simulink model "Att_project_simulink"  (R2022b)
settings: Solver=ode8  StartTime=0.0  StopTime=5000  FixedStep=0.5  RelTol=1e-9  AbsTol=1e-9
values from neighbouring files (symbols this model uses):
  A_R = A_R_BL * ALN_R    [Attitude_proj.m]
  A_T = A_R_BL    [Attitude_proj.m]
  accuracy_earth = deg2rad(10/60)    [Attitude_proj.m]
  accuracy_mag = deg2rad(300/60)    [Attitude_proj.m]
  Cd = 2.3    [Attitude_proj.m]
  I = [Ix 0 0; 0 Iy 0 ; 0 0 Iz]    [Attitude_proj.m]
  Ix = 0.07    [Attitude_proj.m]
  Iy = 0.0504    [Attitude_proj.m]
  Iz = 0.0109    [Attitude_proj.m]
  kd_detum = 2 .* kp_detum    [Attitude_proj.m]
  kd_slew = 2 * kp_slew    [Attitude_proj.m]
  kd_track = kd_detum    [Attitude_proj.m]
  kp_detum = [0.00008 0.0005 0.0005]    [Attitude_proj.m]
  kp_slew = [0.0005 0.0004 0.0004]    [Attitude_proj.m]
  kp_track = kp_detum    [Attitude_proj.m]
  Kx = (Iy-Iz)/Ix    (= 0.564285714286)    [Attitude_proj.m]
  Ky = (Iz-Ix)/Iy    (= -1.17261904762)    [Attitude_proj.m]
  Kz = (Ix-Iy)/Iz    (= 1.79816513761)    [Attitude_proj.m]
  m_para = [0.03;0.04;0.05]    [Attitude_proj.m]
  ortog = (1/3 * deg2rad(1)^2)    [Attitude_proj.m]
  P = Fe/c    (= 4.52980041279e-06)    [Attitude_proj.m]
  q_r = [q1r q2r q3r q4r]    [Attitude_proj.m]
  rho_d_main = 0.1    [Attitude_proj.m]
  rho_d_panel = 0.1    [Attitude_proj.m]
  rho_s_main = 0.5    [Attitude_proj.m]
  rho_s_panel = 0.1    [Attitude_proj.m]
  Rs = 147098074    [Attitude_proj.m]
  w0x = 0.0001    [Attitude_proj.m]
  w0y = orbit.n + 0.005    [Attitude_proj.m]
  w0z = 0.0002    [Attitude_proj.m]
  w_track = [0; orbit.n ; 0]    [Attitude_proj.m]
  zero_w = [ 0; 0; 0]    [Attitude_proj.m]
undefined symbols (not defined in the file or in its folder): body, DiscIntNeverNeededParam, g, h, K, k2, magnitude, orbit, phi0, psi0, theta0, thrus
libraries: vrlib x60, matrix_library x7, simulink x4, sharedutil x4, simulink_extras x2, cstblocks x1, aerolibconvert2 x1, sharedtransform x1
(part 2 of 2)

== system Att_project_simulink/Kynematics/Quaternions ==
  wB : Inport
  Demux : Demux  Outputs=3
  Determinant of 3x3 Matrix : sharedutil/Determinant of 3x3 Matrix  aMode=aMode
  Gain : Gain  Gain=-1
  Gain1 : Gain  Gain=-1
  Gain2 : Gain  Gain=-1
  Gain3 : Gain  Gain=0.5
  Ground{,1..3} (4 alike) : Ground
  Integrator : Integrator  InitialCondition=q_r
  MatrixMultiply : Product  Multiplication=Matrix(*)
  Quaternions to Direction Cosine Matrix : sharedtransform/Quaternions to  Direction Cosine Matrix  aMode=aMode
  Reshape : Reshape  OutputDimensionality=Customize  OutputDimensions=[4,4]
  Scope : Scope
  Scope1 : Scope
  Scope2 : Scope
  To Workspace : ToWorkspace  VariableName=quaternions  SaveFormat=Timeseries  SampleTime=-1
  Vector Concatenate : Concatenate  NumInputs=16
  q(t) : Outport
  tag scope: q=global
  wires:
  wB/1 -> Demux/1
  Ground3/1 -> Vector Concatenate/1
  Ground2/1 -> Vector Concatenate/6
  Ground1/1 -> Vector Concatenate/16
  Ground/1 -> Vector Concatenate/11
  Demux/1 -> Vector Concatenate/13, Vector Concatenate/10, Gain/1  "w_x"
  Demux/2 -> Vector Concatenate/3, Vector Concatenate/14, Gain1/1  "w_y"
  Demux/3 -> Vector Concatenate/5, Gain2/1, Vector Concatenate/15  "w_z"
  Gain2/1 -> Vector Concatenate/12, Vector Concatenate/2
  Gain/1 -> Vector Concatenate/4, Vector Concatenate/7
  Gain1/1 -> Vector Concatenate/9, Vector Concatenate/8
  Vector Concatenate/1 -> Reshape/1
  Reshape/1 -> Gain3/1  "Omega"
  Gain3/1 -> MatrixMultiply/1
  MatrixMultiply/1 -> Integrator/1
  Integrator/1 -> q(t)/1, Quaternions to Direction Cosine Matrix/1, [q], To Workspace/1, Scope/1, MatrixMultiply/2  "q(t)"
  Quaternions to Direction Cosine Matrix/1 -> Determinant of 3x3 Matrix/1, Scope1/1
  Determinant of 3x3 Matrix/1 -> Scope2/1

== system Att_project_simulink/Attitude determination/Triad Method/Error ==
  A_err : Inport
  Acos2 : Trigonometry  Operator=acos
  Constant6 : Constant
  Extract Diagonal3 : matrix_library/Extract Diagonal
      settings: LibrarySourceBlock=|
      | simulink/Matrix
      | Operations/Extract Diagonal
  Gain2 : Gain  Gain=0.5
  Radians to Degrees2 : simulink_extras/Transformations/Radians to Degrees
  Sum of Elements3 : Sum  Inputs=+
  Sum7 : Sum  Inputs=|+-
  error : Outport
  wires:
  Extract Diagonal3/1 -> Sum of Elements3/1
  Acos2/1 -> Radians to Degrees2/1
  Sum of Elements3/1 -> Sum7/1
  Radians to Degrees2/1 -> error/1
  A_err/1 -> Extract Diagonal3/1
  Sum7/1 -> Gain2/1
  Constant6/1 -> Sum7/2
  Gain2/1 -> Acos2/1

== system Att_project_simulink/Attitude determination/Triad Method/Error1 ==
  Id : Inport
  Acos2 : Trigonometry  Operator=acos
  Constant6 : Constant
  Extract Diagonal3 : matrix_library/Extract Diagonal
      settings: LibrarySourceBlock=|
      | simulink/Matrix
      | Operations/Extract Diagonal
  Gain2 : Gain  Gain=0.5
  Radians to Degrees2 : simulink_extras/Transformations/Radians to Degrees
  Sum of Elements3 : Sum  Inputs=+
  Sum7 : Sum  Inputs=|+-
  error : Outport
  wires:
  Gain2/1 -> Acos2/1
  Constant6/1 -> Sum7/2
  Sum7/1 -> Gain2/1
  Id/1 -> Extract Diagonal3/1
  Radians to Degrees2/1 -> error/1
  Sum of Elements3/1 -> Sum7/1
  Acos2/1 -> Radians to Degrees2/1
  Extract Diagonal3/1 -> Sum of Elements3/1

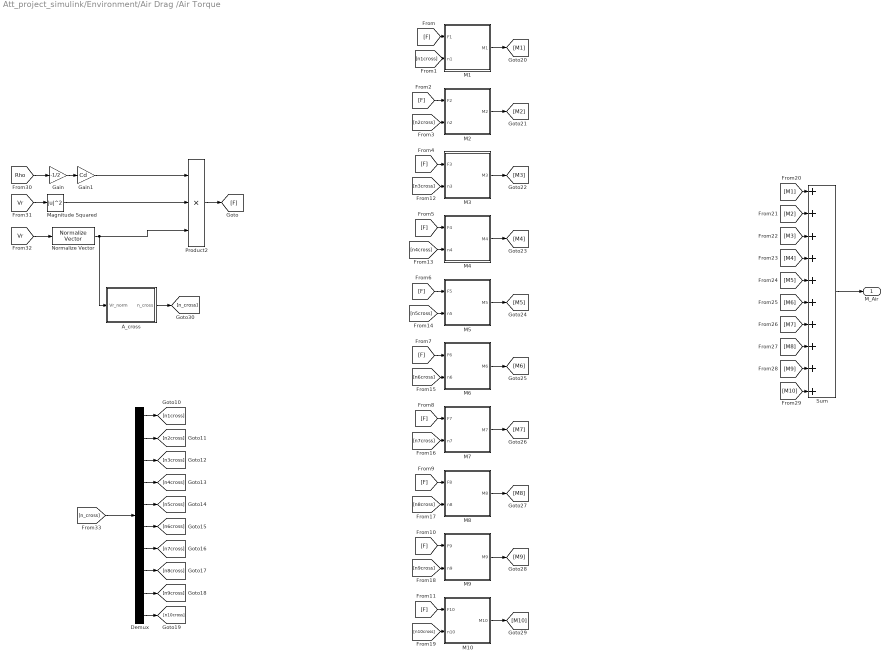
== system Att_project_simulink/Environment/Air Drag /Air Torque ==
  A_cross : Subsystem
  Demux : Demux  Outputs=10
  Gain : Gain  Gain=-1/2
  Gain1 : Gain  Gain=Cd
  M1 : Subsystem
  M10 : Subsystem
  M2 : Subsystem
  M3 : Subsystem
  M4 : Subsystem
  M5 : Subsystem
  M6 : Subsystem
  M7 : Subsystem
  M8 : Subsystem
  M9 : Subsystem
  Magnitude Squared : Math  Operator=magnitude^2
  Normalize Vector : vrlib/Utilities/Normalize Vector  maxzero=0
  Product2 : Product  Inputs=3
  Sum : Sum  Inputs=++++++++++
  M_Air : Outport
  wires:
  [n_cross] -> Demux/1
  Demux/1 -> [n1cross]
  Demux/2 -> [n2cross]
  Demux/3 -> [n3cross]
  Demux/4 -> [n4cross]
  Demux/5 -> [n5cross]
  Demux/6 -> [n6cross]
  Demux/7 -> [n7cross]
  Demux/8 -> [n8cross]
  Demux/9 -> [n9cross]
  Demux/10 -> [n10cross]
  [F] -> M1/1(F1)
  [n1cross] -> M1/2(n1)
  [F] -> M2/1(F2)
  [F] -> M10/1(F10)
  [F] -> M9/1(F9)
  [F] -> M8/1(F8)
  [F] -> M7/1(F7)
  [F] -> M6/1(F6)
  [F] -> M5/1(F5)
  [F] -> M4/1(F4)
  [F] -> M3/1(F3)
  [n3cross] -> M3/2(n3)
  [n4cross] -> M4/2(n4)
  [n5cross] -> M5/2(n5)
  [n6cross] -> M6/2(n6)
  [n7cross] -> M7/2(n7)
  [n8cross] -> M8/2(n8)
  [n9cross] -> M9/2(n9)
  [n10cross] -> M10/2(n10)
  [n2cross] -> M2/2(n2)
  M1/1(M1) -> [M1]
  M2/1(M2) -> [M2]
  M3/1(M3) -> [M3]
  M4/1(M4) -> [M4]
  M5/1(M5) -> [M5]
  M6/1(M6) -> [M6]
  M7/1(M7) -> [M7]
  M8/1(M8) -> [M8]
  M9/1(M9) -> [M9]
  M10/1(M10) -> [M10]
  [M1] -> Sum/1
  [M2] -> Sum/2
  [M3] -> Sum/3
  [M4] -> Sum/4
  [M5] -> Sum/5
  [M6] -> Sum/6
  [M7] -> Sum/7
  [M8] -> Sum/8
  [M9] -> Sum/9
  [M10] -> Sum/10
  Sum/1 -> M_Air/1
  [Rho] -> Gain/1
  A_cross/1(n_cross) -> [n_cross]
  Gain/1 -> Gain1/1
  Gain1/1 -> Product2/1
  Magnitude Squared/1 -> Product2/2
  [Vr] -> Magnitude Squared/1
  Product2/1 -> [F]
  [Vr] -> Normalize Vector/1
  Normalize Vector/1 -> A_cross/1(Vr_norm), Product2/3

== system Att_project_simulink/Environment/Magnetif Field Model/Ground Track ==
  Rn : Inport
  ThetaG0 : Inport  Port=2
  t : Inport  Port=3
  W_E : Inport  Port=4
  t0 : Inport  Port=5
  Asin : Trigonometry  Operator=asin
  Atan2 : Trigonometry  Operator=atan2
  Divide : Product  Inputs=*/
  Math Function : Math  Operator=square  SignedPower=on
  Math Function1 : Math  Operator=sqrt  SignedPower=on
  Product : Product
  Selector : Selector  InputPortWidth=3  IndexOptions=Index vector (dialog)  Indices=[3]  OutputSizes=1
  Selector1 : Selector  InputPortWidth=3  IndexOptions=Index vector (dialog)  Indices=[2]  OutputSizes=1
  Selector2 : Selector  InputPortWidth=3  IndexOptions=Index vector (dialog)  Indices=[1 ]  OutputSizes=1
  Sum : Sum  Inputs=|+-
  Sum of Elements : Sum  Inputs=+
  Sum1 : Sum  Inputs=|++
  Sum2 : Sum  Inputs=|+-
  Lon : Outport
  Lat : Outport  Port=2
  R_norm : Outport  Port=3
  wires:
  Rn/1 -> Selector2/1, Selector1/1, Math Function/1, Selector/1
  Selector/1 -> Divide/1
  Math Function1/1 -> R_norm/1, Divide/2
  Divide/1 -> Asin/1
  Asin/1 -> Lat/1
  Selector1/1 -> Atan2/1
  Selector2/1 -> Atan2/2
  t/1 -> Sum/1
  t0/1 -> Sum/2
  Sum/1 -> Product/1
  W_E/1 -> Product/2
  Product/1 -> Sum1/1
  ThetaG0/1 -> Sum1/2
  Sum1/1 -> Sum2/2  "ThetaG"
  Atan2/1 -> Sum2/1
  Sum2/1 -> Lon/1
  Math Function/1 -> Sum of Elements/1
  Sum of Elements/1 -> Math Function1/1

== system Att_project_simulink/Environment/SRP/F1 ==
  In1 : Inport
  Input : Inport  Port=2
  Constant : Constant  Value=-P
  Constant1 : Constant  Value=body.A1
  Constant2 : Constant
  Constant3 : Constant  Value=body.r1
  Constant6 : Constant  Value=rho_s_main
  Constant7 : Constant  Value=(2/3)*rho_d_main
  Cross Product : vrlib/Utilities/Cross Product
  Dot Product : DotProduct  OutDataTypeStr=Inherit: Inherit via internal rule
  Dot Product1 : DotProduct  OutDataTypeStr=Inherit: Inherit via internal rule
  Gain3 : Gain  Gain=2*rho_s_main
  Normalize Vector : vrlib/Utilities/Normalize Vector  maxzero=0
  Normalize Vector1 : vrlib/Utilities/Normalize Vector  maxzero=0
  Normalize Vector2 : vrlib/Utilities/Normalize Vector  maxzero=0
  Product : Product  Inputs=3
  Product1 : Product
  Product2 : Product
  Product3 : Product
  Sum : Sum  Inputs=+-
  Sum1 : Sum
  Sum2 : Sum  Inputs=|++
  Switch : Switch  Criteria=u2 > Threshold  SaturateOnIntegerOverflow=off  InputSameDT=off
  Zero : Constant  Value=0  OutDataTypeStr=Inherit: Inherit via back propagation
  T1 : Outport
  wires:
  Dot Product/1 -> Product/3
  Sum1/1 -> Product3/2
  Product2/1 -> Sum1/2
  Constant2/1 -> Sum/1
  [n1] -> Dot Product1/2
  Constant6/1 -> Sum/2
  Sum2/1 -> Product2/2
  Gain3/1 -> Sum2/1
  Constant7/1 -> Sum2/2
  Product1/1 -> Sum1/1
  Sum/1 -> Product1/1
  [n1] -> Product2/1
  Product/1 -> Product3/1
  Constant1/1 -> Product/2
  [n1] -> Dot Product/2
  Constant/1 -> Product/1
  In1/1 -> [n1]
  Input/1 -> [Sb]
  Dot Product1/1 -> [Sb_dot_N1], Gain3/1
  [Sb_dot_N1] -> Switch/2
  Zero/1 -> Switch/3
  Product3/1 -> Switch/1
  Switch/1 -> Cross Product/1
  Constant3/1 -> Cross Product/2
  Cross Product/1 -> T1/1
  [Sb] -> Normalize Vector/1
  Normalize Vector/1 -> Dot Product/1
  [Sb] -> Normalize Vector1/1
  Normalize Vector1/1 -> Product1/2
  [Sb] -> Normalize Vector2/1
  Normalize Vector2/1 -> Dot Product1/1

== system Att_project_simulink/Environment/SRP/F10 ==
  In1 : Inport
  In2 : Inport  Port=2
  Constant10 : Constant
  Constant11 : Constant  Value=rho_s_panel
  Constant12 : Constant  Value=(2/3)*rho_d_panel
  Constant3 : Constant  Value=body.r10
  Constant8 : Constant  Value=-P
  Constant9 : Constant  Value=body.A10
  Cross Product : vrlib/Utilities/Cross Product
  Dot Product2 : DotProduct  OutDataTypeStr=Inherit: Inherit via internal rule
  Dot Product3 : DotProduct  OutDataTypeStr=Inherit: Inherit via internal rule
  Gain4 : Gain  Gain=2*rho_s_panel
  Normalize Vector : vrlib/Utilities/Normalize Vector  maxzero=0
  Normalize Vector1 : vrlib/Utilities/Normalize Vector  maxzero=0
  Normalize Vector2 : vrlib/Utilities/Normalize Vector  maxzero=0
  Product3 : Product
  Product4 : Product  Inputs=3
  Product5 : Product
  Product6 : Product
  Sum3 : Sum  Inputs=+-
  Sum4 : Sum
  Sum5 : Sum  Inputs=|++
  Switch : Switch  Criteria=u2 > Threshold  SaturateOnIntegerOverflow=off  InputSameDT=off
  Zero : Constant  Value=0  OutDataTypeStr=Inherit: Inherit via back propagation
  T10 : Outport
  wires:
  Product6/1 -> Sum4/2
  Constant9/1 -> Product4/2
  Gain4/1 -> Sum5/1
  Dot Product2/1 -> Product4/3
  [n10] -> Dot Product2/2
  Sum3/1 -> Product5/1
  Constant11/1 -> Sum3/2
  Constant8/1 -> Product4/1
  Sum5/1 -> Product6/2
  Product4/1 -> Product3/1
  Constant12/1 -> Sum5/2
  [n10] -> Product6/1
  Product5/1 -> Sum4/1
  [n10] -> Dot Product3/2
  Dot Product3/1 -> [Sb_dot_N10], Gain4/1
  Constant10/1 -> Sum3/1
  Sum4/1 -> Product3/2
  In1/1 -> [n10]
  In2/1 -> [Sb]
  Cross Product/1 -> T10/1
  Constant3/1 -> Cross Product/2
  Product3/1 -> Switch/1
  [Sb_dot_N10] -> Switch/2
  Switch/1 -> Cross Product/1
  Zero/1 -> Switch/3
  [Sb] -> Normalize Vector/1
  Normalize Vector/1 -> Dot Product2/1
  [Sb] -> Normalize Vector1/1
  Normalize Vector1/1 -> Product5/2
  [Sb] -> Normalize Vector2/1
  Normalize Vector2/1 -> Dot Product3/1

== system Att_project_simulink/Environment/SRP/F2 ==
  In1 : Inport
  In2 : Inport  Port=2
  Constant10 : Constant
  Constant11 : Constant  Value=rho_s_main
  Constant12 : Constant  Value=(2/3)*rho_d_main
  Constant3 : Constant  Value=body.r2
  Constant8 : Constant  Value=-P
  Constant9 : Constant  Value=body.A2
  Cross Product : vrlib/Utilities/Cross Product
  Dot Product2 : DotProduct  OutDataTypeStr=Inherit: Inherit via internal rule
  Dot Product3 : DotProduct  OutDataTypeStr=Inherit: Inherit via internal rule
  Gain4 : Gain  Gain=2*rho_s_main
  Normalize Vector : vrlib/Utilities/Normalize Vector  maxzero=0
  Normalize Vector1 : vrlib/Utilities/Normalize Vector  maxzero=0
  Normalize Vector2 : vrlib/Utilities/Normalize Vector  maxzero=0
  Product3 : Product
  Product4 : Product  Inputs=3
  Product5 : Product
  Product6 : Product
  Sum3 : Sum  Inputs=+-
  Sum4 : Sum
  Sum5 : Sum  Inputs=|++
  Switch : Switch  Criteria=u2 > Threshold  SaturateOnIntegerOverflow=off  InputSameDT=off
  Zero : Constant  Value=0  OutDataTypeStr=Inherit: Inherit via back propagation
  T2 : Outport
  wires:
  Product6/1 -> Sum4/2
  Constant9/1 -> Product4/2
  Gain4/1 -> Sum5/1
  Dot Product2/1 -> Product4/3
  [n2] -> Dot Product2/2
  Sum3/1 -> Product5/1
  Constant11/1 -> Sum3/2
  Constant8/1 -> Product4/1
  Sum5/1 -> Product6/2
  Product4/1 -> Product3/1
  Constant12/1 -> Sum5/2
  [n2] -> Product6/1
  Product5/1 -> Sum4/1
  [n2] -> Dot Product3/2
  Dot Product3/1 -> [Sb_dot_N2], Gain4/1
  Constant10/1 -> Sum3/1
  Sum4/1 -> Product3/2
  In1/1 -> [n2]
  In2/1 -> [Sb]
  Cross Product/1 -> T2/1
  Constant3/1 -> Cross Product/2
  Product3/1 -> Switch/1
  [Sb_dot_N2] -> Switch/2
  Switch/1 -> Cross Product/1
  Zero/1 -> Switch/3
  [Sb] -> Normalize Vector/1
  Normalize Vector/1 -> Dot Product2/1
  [Sb] -> Normalize Vector1/1
  Normalize Vector1/1 -> Product5/2
  [Sb] -> Normalize Vector2/1
  Normalize Vector2/1 -> Dot Product3/1

== system Att_project_simulink/Environment/SRP/F3 ==
  In1 : Inport
  In2 : Inport  Port=2
  Constant10 : Constant
  Constant11 : Constant  Value=rho_s_main
  Constant12 : Constant  Value=(2/3)*rho_d_main
  Constant3 : Constant  Value=body.r3
  Constant8 : Constant  Value=-P
  Constant9 : Constant  Value=body.A3
  Cross Product : vrlib/Utilities/Cross Product
  Dot Product2 : DotProduct  OutDataTypeStr=Inherit: Inherit via internal rule
  Dot Product3 : DotProduct  OutDataTypeStr=Inherit: Inherit via internal rule
  Gain4 : Gain  Gain=2*rho_s_main
  Normalize Vector : vrlib/Utilities/Normalize Vector  maxzero=0
  Normalize Vector1 : vrlib/Utilities/Normalize Vector  maxzero=0
  Normalize Vector2 : vrlib/Utilities/Normalize Vector  maxzero=0
  Product3 : Product
  Product4 : Product  Inputs=3
  Product5 : Product
  Product6 : Product
  Sum3 : Sum  Inputs=+-
  Sum4 : Sum
  Sum5 : Sum  Inputs=|++
  Switch : Switch  Criteria=u2 > Threshold  SaturateOnIntegerOverflow=off  InputSameDT=off
  Zero : Constant  Value=0  OutDataTypeStr=Inherit: Inherit via back propagation
  T3 : Outport
  wires:
  Product6/1 -> Sum4/2
  Constant9/1 -> Product4/2
  Gain4/1 -> Sum5/1
  Dot Product2/1 -> Product4/3
  [n3] -> Dot Product2/2
  Sum3/1 -> Product5/1
  Constant11/1 -> Sum3/2
  Constant8/1 -> Product4/1
  Sum5/1 -> Product6/2
  Product4/1 -> Product3/1
  Constant12/1 -> Sum5/2
  [n3] -> Product6/1
  Product5/1 -> Sum4/1
  [n3] -> Dot Product3/2
  Dot Product3/1 -> [Sb_dot_N3], Gain4/1
  Constant10/1 -> Sum3/1
  Sum4/1 -> Product3/2
  In1/1 -> [n3]
  In2/1 -> [Sb]
  Cross Product/1 -> T3/1
  Constant3/1 -> Cross Product/2
  Product3/1 -> Switch/1
  [Sb_dot_N3] -> Switch/2
  Switch/1 -> Cross Product/1
  Zero/1 -> Switch/3
  Normalize Vector/1 -> Dot Product2/1
  [Sb] -> Normalize Vector/1
  Normalize Vector1/1 -> Product5/2
  [Sb] -> Normalize Vector1/1
  [Sb] -> Normalize Vector2/1
  Normalize Vector2/1 -> Dot Product3/1

== system Att_project_simulink/Environment/SRP/F4 ==
  In1 : Inport
  In2 : Inport  Port=2
  Constant10 : Constant
  Constant11 : Constant  Value=rho_s_main
  Constant12 : Constant  Value=(2/3)*rho_d_main
  Constant3 : Constant  Value=body.r4
  Constant8 : Constant  Value=-P
  Constant9 : Constant  Value=body.A4
  Cross Product : vrlib/Utilities/Cross Product
  Dot Product2 : DotProduct  OutDataTypeStr=Inherit: Inherit via internal rule
  Dot Product3 : DotProduct  OutDataTypeStr=Inherit: Inherit via internal rule
  Gain4 : Gain  Gain=2*rho_s_main
  Normalize Vector : vrlib/Utilities/Normalize Vector  maxzero=0
  Normalize Vector1 : vrlib/Utilities/Normalize Vector  maxzero=0
  Normalize Vector2 : vrlib/Utilities/Normalize Vector  maxzero=0
  Product3 : Product
  Product4 : Product  Inputs=3
  Product5 : Product
  Product6 : Product
  Sum3 : Sum  Inputs=+-
  Sum4 : Sum
  Sum5 : Sum  Inputs=|++
  Switch : Switch  Criteria=u2 > Threshold  SaturateOnIntegerOverflow=off  InputSameDT=off
  Zero : Constant  Value=0  OutDataTypeStr=Inherit: Inherit via back propagation
  T4 : Outport
  wires:
  Product6/1 -> Sum4/2
  Constant9/1 -> Product4/2
  Gain4/1 -> Sum5/1
  Dot Product2/1 -> Product4/3
  [n4] -> Dot Product2/2
  Sum3/1 -> Product5/1
  Constant11/1 -> Sum3/2
  Constant8/1 -> Product4/1
  Sum5/1 -> Product6/2
  Product4/1 -> Product3/1
  Constant12/1 -> Sum5/2
  [n4] -> Product6/1
  Product5/1 -> Sum4/1
  [n4] -> Dot Product3/2
  Dot Product3/1 -> [Sb_dot_N4], Gain4/1
  Constant10/1 -> Sum3/1
  Sum4/1 -> Product3/2
  In1/1 -> [n4]
  In2/1 -> [Sb]
  Cross Product/1 -> T4/1
  Constant3/1 -> Cross Product/2
  Product3/1 -> Switch/1
  [Sb_dot_N4] -> Switch/2
  Switch/1 -> Cross Product/1
  Zero/1 -> Switch/3
  [Sb] -> Normalize Vector/1
  Normalize Vector/1 -> Dot Product2/1
  [Sb] -> Normalize Vector1/1
  Normalize Vector1/1 -> Product5/2
  [Sb] -> Normalize Vector2/1
  Normalize Vector2/1 -> Dot Product3/1

== system Att_project_simulink/Environment/SRP/F5 ==
  In1 : Inport
  In2 : Inport  Port=2
  Constant10 : Constant
  Constant11 : Constant  Value=rho_s_main
  Constant12 : Constant  Value=(2/3)*rho_d_main
  Constant3 : Constant  Value=body.r5
  Constant8 : Constant  Value=-P
  Constant9 : Constant  Value=body.A5
  Cross Product : vrlib/Utilities/Cross Product
  Dot Product2 : DotProduct  OutDataTypeStr=Inherit: Inherit via internal rule
  Dot Product3 : DotProduct  OutDataTypeStr=Inherit: Inherit via internal rule
  Gain4 : Gain  Gain=2*rho_s_main
  Normalize Vector : vrlib/Utilities/Normalize Vector  maxzero=0
  Normalize Vector1 : vrlib/Utilities/Normalize Vector  maxzero=0
  Normalize Vector2 : vrlib/Utilities/Normalize Vector  maxzero=0
  Product3 : Product
  Product4 : Product  Inputs=3
  Product5 : Product
  Product6 : Product
  Sum3 : Sum  Inputs=+-
  Sum4 : Sum
  Sum5 : Sum  Inputs=|++
  Switch : Switch  Criteria=u2 > Threshold  SaturateOnIntegerOverflow=off  InputSameDT=off
  Zero : Constant  Value=0  OutDataTypeStr=Inherit: Inherit via back propagation
  T5 : Outport
  wires:
  Product6/1 -> Sum4/2
  Constant9/1 -> Product4/2
  Gain4/1 -> Sum5/1
  Dot Product2/1 -> Product4/3
  [n5] -> Dot Product2/2
  Sum3/1 -> Product5/1
  Constant11/1 -> Sum3/2
  Constant8/1 -> Product4/1
  Sum5/1 -> Product6/2
  Product4/1 -> Product3/1
  Constant12/1 -> Sum5/2
  [n5] -> Product6/1
  Product5/1 -> Sum4/1
  [n5] -> Dot Product3/2
  Dot Product3/1 -> [Sb_dot_N5], Gain4/1
  Constant10/1 -> Sum3/1
  Sum4/1 -> Product3/2
  In1/1 -> [n5]
  In2/1 -> [Sb]
  Cross Product/1 -> T5/1
  Constant3/1 -> Cross Product/2
  Product3/1 -> Switch/1
  [Sb_dot_N5] -> Switch/2
  Switch/1 -> Cross Product/1
  Zero/1 -> Switch/3
  [Sb] -> Normalize Vector/1
  Normalize Vector/1 -> Dot Product2/1
  [Sb] -> Normalize Vector1/1
  Normalize Vector1/1 -> Product5/2
  [Sb] -> Normalize Vector2/1
  Normalize Vector2/1 -> Dot Product3/1

== system Att_project_simulink/Environment/SRP/F6 ==
  In1 : Inport
  In2 : Inport  Port=2
  Constant10 : Constant
  Constant11 : Constant  Value=rho_s_main
  Constant12 : Constant  Value=(2/3)*rho_d_main
  Constant3 : Constant  Value=body.r6
  Constant8 : Constant  Value=-P
  Constant9 : Constant  Value=body.A6
  Cross Product : vrlib/Utilities/Cross Product
  Dot Product2 : DotProduct  OutDataTypeStr=Inherit: Inherit via internal rule
  Dot Product3 : DotProduct  OutDataTypeStr=Inherit: Inherit via internal rule
  Gain4 : Gain  Gain=2*rho_s_main
  Normalize Vector : vrlib/Utilities/Normalize Vector  maxzero=0
  Normalize Vector1 : vrlib/Utilities/Normalize Vector  maxzero=0
  Normalize Vector2 : vrlib/Utilities/Normalize Vector  maxzero=0
  Product3 : Product
  Product4 : Product  Inputs=3
  Product5 : Product
  Product6 : Product
  Sum3 : Sum  Inputs=+-
  Sum4 : Sum
  Sum5 : Sum  Inputs=|++
  Switch : Switch  Criteria=u2 > Threshold  SaturateOnIntegerOverflow=off  InputSameDT=off
  Zero : Constant  Value=0  OutDataTypeStr=Inherit: Inherit via back propagation
  T6 : Outport
  wires:
  Product6/1 -> Sum4/2
  Constant9/1 -> Product4/2
  Gain4/1 -> Sum5/1
  Dot Product2/1 -> Product4/3
  [n6] -> Dot Product2/2
  Sum3/1 -> Product5/1
  Constant11/1 -> Sum3/2
  Constant8/1 -> Product4/1
  Sum5/1 -> Product6/2
  Product4/1 -> Product3/1
  Constant12/1 -> Sum5/2
  [n6] -> Product6/1
  Product5/1 -> Sum4/1
  [n6] -> Dot Product3/2
  Dot Product3/1 -> [Sb_dot_N6], Gain4/1
  Constant10/1 -> Sum3/1
  Sum4/1 -> Product3/2
  In1/1 -> [n6]
  In2/1 -> [Sb]
  Cross Product/1 -> T6/1
  Constant3/1 -> Cross Product/2
  Product3/1 -> Switch/1
  [Sb_dot_N6] -> Switch/2
  Switch/1 -> Cross Product/1
  Zero/1 -> Switch/3
  Normalize Vector/1 -> Dot Product2/1
  [Sb] -> Normalize Vector/1
  [Sb] -> Normalize Vector1/1
  Normalize Vector1/1 -> Product5/2
  [Sb] -> Normalize Vector2/1
  Normalize Vector2/1 -> Dot Product3/1

== system Att_project_simulink/Environment/SRP/F7 ==
  In1 : Inport
  In2 : Inport  Port=2
  Constant10 : Constant
  Constant11 : Constant  Value=rho_s_panel
  Constant12 : Constant  Value=(2/3)*rho_d_panel
  Constant3 : Constant  Value=body.r7
  Constant8 : Constant  Value=-P
  Constant9 : Constant  Value=body.A7
  Cross Product : vrlib/Utilities/Cross Product
  Dot Product2 : DotProduct  OutDataTypeStr=Inherit: Inherit via internal rule
  Dot Product3 : DotProduct  OutDataTypeStr=Inherit: Inherit via internal rule
  Gain4 : Gain  Gain=2*rho_s_panel
  Normalize Vector : vrlib/Utilities/Normalize Vector  maxzero=0
  Normalize Vector1 : vrlib/Utilities/Normalize Vector  maxzero=0
  Normalize Vector2 : vrlib/Utilities/Normalize Vector  maxzero=0
  Product3 : Product
  Product4 : Product  Inputs=3
  Product5 : Product
  Product6 : Product
  Sum3 : Sum  Inputs=+-
  Sum4 : Sum
  Sum5 : Sum  Inputs=|++
  Switch : Switch  Criteria=u2 > Threshold  SaturateOnIntegerOverflow=off  InputSameDT=off
  Zero : Constant  Value=0  OutDataTypeStr=Inherit: Inherit via back propagation
  T7 : Outport
  wires:
  Product6/1 -> Sum4/2
  Constant9/1 -> Product4/2
  Gain4/1 -> Sum5/1
  Dot Product2/1 -> Product4/3
  [n7] -> Dot Product2/2
  Sum3/1 -> Product5/1
  Constant11/1 -> Sum3/2
  Constant8/1 -> Product4/1
  Sum5/1 -> Product6/2
  Product4/1 -> Product3/1
  Constant12/1 -> Sum5/2
  [n7] -> Product6/1
  Product5/1 -> Sum4/1
  [n7] -> Dot Product3/2
  Dot Product3/1 -> [Sb_dot_N7], Gain4/1
  Constant10/1 -> Sum3/1
  Sum4/1 -> Product3/2
  In2/1 -> [Sb]
  In1/1 -> [n7]
  Cross Product/1 -> T7/1
  Constant3/1 -> Cross Product/2
  Product3/1 -> Switch/1
  [Sb_dot_N7] -> Switch/2
  Switch/1 -> Cross Product/1
  Zero/1 -> Switch/3
  [Sb] -> Normalize Vector/1
  Normalize Vector/1 -> Dot Product2/1
  [Sb] -> Normalize Vector1/1
  Normalize Vector1/1 -> Product5/2
  [Sb] -> Normalize Vector2/1
  Normalize Vector2/1 -> Dot Product3/1

== system Att_project_simulink/Environment/SRP/F8 ==
  In1 : Inport
  In2 : Inport  Port=2
  Constant10 : Constant
  Constant11 : Constant  Value=rho_s_panel
  Constant12 : Constant  Value=(2/3)*rho_d_panel
  Constant3 : Constant  Value=body.r8
  Constant8 : Constant  Value=-P
  Constant9 : Constant  Value=body.A8
  Cross Product : vrlib/Utilities/Cross Product
  Dot Product2 : DotProduct  OutDataTypeStr=Inherit: Inherit via internal rule
  Dot Product3 : DotProduct  OutDataTypeStr=Inherit: Inherit via internal rule
  Gain4 : Gain  Gain=2*rho_s_panel
  Normalize Vector : vrlib/Utilities/Normalize Vector  maxzero=0
  Normalize Vector1 : vrlib/Utilities/Normalize Vector  maxzero=0
  Normalize Vector2 : vrlib/Utilities/Normalize Vector  maxzero=0
  Product3 : Product
  Product4 : Product  Inputs=3
  Product5 : Product
  Product6 : Product
  Sum3 : Sum  Inputs=+-
  Sum4 : Sum
  Sum5 : Sum  Inputs=|++
  Switch : Switch  Criteria=u2 > Threshold  SaturateOnIntegerOverflow=off  InputSameDT=off
  Zero : Constant  Value=0  OutDataTypeStr=Inherit: Inherit via back propagation
  T8 : Outport
  wires:
  Product6/1 -> Sum4/2
  Constant9/1 -> Product4/2
  Gain4/1 -> Sum5/1
  Dot Product2/1 -> Product4/3
  [n8] -> Dot Product2/2
  Sum3/1 -> Product5/1
  Constant11/1 -> Sum3/2
  Constant8/1 -> Product4/1
  Sum5/1 -> Product6/2
  Product4/1 -> Product3/1
  Constant12/1 -> Sum5/2
  [n8] -> Product6/1
  Product5/1 -> Sum4/1
  [n8] -> Dot Product3/2
  Dot Product3/1 -> [Sb_dot_N8], Gain4/1
  Constant10/1 -> Sum3/1
  Sum4/1 -> Product3/2
  In1/1 -> [n8]
  In2/1 -> [Sb]
  Cross Product/1 -> T8/1
  Constant3/1 -> Cross Product/2
  Product3/1 -> Switch/1
  [Sb_dot_N8] -> Switch/2
  Switch/1 -> Cross Product/1
  Zero/1 -> Switch/3
  [Sb] -> Normalize Vector/1
  Normalize Vector/1 -> Dot Product2/1
  [Sb] -> Normalize Vector1/1
  Normalize Vector1/1 -> Product5/2
  [Sb] -> Normalize Vector2/1
  Normalize Vector2/1 -> Dot Product3/1

== system Att_project_simulink/Environment/SRP/F9 ==
  In1 : Inport
  In2 : Inport  Port=2
  Constant10 : Constant
  Constant11 : Constant  Value=rho_s_panel
  Constant12 : Constant  Value=(2/3)*rho_d_panel
  Constant3 : Constant  Value=body.r9
  Constant8 : Constant  Value=-P
  Constant9 : Constant  Value=body.A9
  Cross Product : vrlib/Utilities/Cross Product
  Dot Product2 : DotProduct  OutDataTypeStr=Inherit: Inherit via internal rule
  Dot Product3 : DotProduct  OutDataTypeStr=Inherit: Inherit via internal rule
  Gain4 : Gain  Gain=2*rho_s_panel
  Normalize Vector : vrlib/Utilities/Normalize Vector  maxzero=0
  Normalize Vector1 : vrlib/Utilities/Normalize Vector  maxzero=0
  Normalize Vector2 : vrlib/Utilities/Normalize Vector  maxzero=0
  Product3 : Product
  Product4 : Product  Inputs=3
  Product5 : Product
  Product6 : Product
  Sum3 : Sum  Inputs=+-
  Sum4 : Sum
  Sum5 : Sum  Inputs=|++
  Switch : Switch  Criteria=u2 > Threshold  SaturateOnIntegerOverflow=off  InputSameDT=off
  Zero : Constant  Value=0  OutDataTypeStr=Inherit: Inherit via back propagation
  T9 : Outport
  wires:
  Product6/1 -> Sum4/2
  Constant9/1 -> Product4/2
  Gain4/1 -> Sum5/1
  Dot Product2/1 -> Product4/3
  [n9] -> Dot Product2/2
  Sum3/1 -> Product5/1
  Constant11/1 -> Sum3/2
  Constant8/1 -> Product4/1
  Sum5/1 -> Product6/2
  Product4/1 -> Product3/1
  Constant12/1 -> Sum5/2
  [n9] -> Product6/1
  Product5/1 -> Sum4/1
  [n9] -> Dot Product3/2
  Dot Product3/1 -> [Sb_dot_N9], Gain4/1
  Constant10/1 -> Sum3/1
  Sum4/1 -> Product3/2
  In1/1 -> [n9]
  In2/1 -> [Sb]
  Cross Product/1 -> T9/1
  Constant3/1 -> Cross Product/2
  Product3/1 -> Switch/1
  [Sb_dot_N9] -> Switch/2
  Switch/1 -> Cross Product/1
  Zero/1 -> Switch/3
  [Sb] -> Normalize Vector/1
  Normalize Vector/1 -> Dot Product2/1
  [Sb] -> Normalize Vector1/1
  Normalize Vector1/1 -> Product5/2
  [Sb] -> Normalize Vector2/1
  Normalize Vector2/1 -> Dot Product3/1

== system Att_project_simulink/Kynematics/DCM/Ortonormalization ==
  In1 : Inport
  Gain6 : Gain  Gain=3/2
  Gain7 : Gain  Gain=1/2
  Product5 : Product  Inputs=3  Multiplication=Matrix(*)
  Sum2 : Sum  Inputs=|+-
  Transpose : Math  Operator=transpose  SignedPower=on
  dcm : Outport
  wires:
  In1/1 -> Gain6/1, Product5/1, Transpose/1, Gain7/1
  Transpose/1 -> Product5/2
  Gain7/1 -> Product5/3
  Gain6/1 -> Sum2/1
  Product5/1 -> Sum2/2
  Sum2/1 -> dcm/1

== system Att_project_simulink/Kynematics/From Quat to DCM/Ortonormalization ==
  In1 : Inport
  Gain6 : Gain  Gain=3/2
  Gain7 : Gain  Gain=1/2
  Product5 : Product  Inputs=3  Multiplication=Matrix(*)
  Sum2 : Sum  Inputs=|+-
  Transpose : Math  Operator=transpose  SignedPower=on
  dcm : Outport
  wires:
  In1/1 -> Gain6/1, Product5/1, Transpose/1, Gain7/1
  Transpose/1 -> Product5/2
  Gain7/1 -> Product5/3
  Gain6/1 -> Sum2/1
  Product5/1 -> Sum2/2
  Sum2/1 -> dcm/1

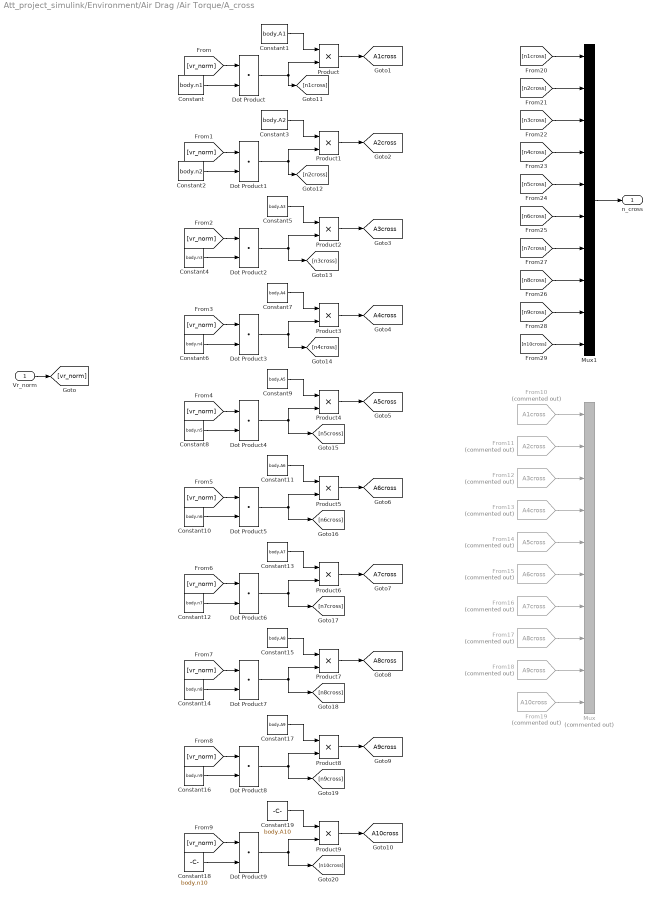
== system Att_project_simulink/Environment/Air Drag /Air Torque/A_cross ==
  Vr_norm : Inport
  Constant : Constant  Value=body.n1
  Constant1 : Constant  Value=body.A1
  Constant10 : Constant  Value=body.n6
  Constant11 : Constant  Value=body.A6
  Constant12 : Constant  Value=body.n7
  Constant13 : Constant  Value=body.A7
  Constant14 : Constant  Value=body.n8
  Constant15 : Constant  Value=body.A8
  Constant16 : Constant  Value=body.n9
  Constant17 : Constant  Value=body.A9
  Constant18 : Constant  Value=body.n10
  Constant19 : Constant  Value=body.A10
  Constant2 : Constant  Value=body.n2
  Constant3 : Constant  Value=body.A2
  Constant4 : Constant  Value=body.n3
  Constant5 : Constant  Value=body.A3
  Constant6 : Constant  Value=body.n4
  Constant7 : Constant  Value=body.A4
  Constant8 : Constant  Value=body.n5
  Constant9 : Constant  Value=body.A5
  Dot Product{,1..9} (10 alike) : DotProduct  OutDataTypeStr=Inherit: Inherit via internal rule
  From10 : From  Commented=on  GotoTag=A1cross
  From11 : From  Commented=on  GotoTag=A2cross
  From12 : From  Commented=on  GotoTag=A3cross
  From13 : From  Commented=on  GotoTag=A4cross
  From14 : From  Commented=on  GotoTag=A5cross
  From15 : From  Commented=on  GotoTag=A6cross
  From16 : From  Commented=on  GotoTag=A7cross
  From17 : From  Commented=on  GotoTag=A8cross
  From18 : From  Commented=on  GotoTag=A9cross
  From19 : From  Commented=on  GotoTag=A10cross
  Mux : Mux  Commented=on  Inputs=10
  Mux1 : Mux  Inputs=10
  Product{,1..9} (10 alike) : Product
  n_cross : Outport
  tag scope: A10cross=global, A1cross=global, A2cross=global, A3cross=global, A4cross=global, A5cross=global, A6cross=global, A7cross=global, A8cross=global, A9cross=global
  wires:
  Vr_norm/1 -> [vr_norm]
  [vr_norm] -> Dot Product/1
  Constant/1 -> Dot Product/2
  Dot Product/1 -> [n1cross], Product/2
  Constant1/1 -> Product/1
  Product/1 -> [A1cross]
  Constant2/1 -> Dot Product1/2
  Constant3/1 -> Product1/1
  Product1/1 -> [A2cross]
  Dot Product1/1 -> [n2cross], Product1/2
  [vr_norm] -> Dot Product1/1
  Constant4/1 -> Dot Product2/2
  Constant5/1 -> Product2/1
  Product2/1 -> [A3cross]
  Dot Product2/1 -> [n3cross], Product2/2
  [vr_norm] -> Dot Product2/1
  Constant6/1 -> Dot Product3/2
  Constant7/1 -> Product3/1
  Product3/1 -> [A4cross]
  Dot Product3/1 -> [n4cross], Product3/2
  [vr_norm] -> Dot Product3/1
  Constant8/1 -> Dot Product4/2
  Constant9/1 -> Product4/1
  Product4/1 -> [A5cross]
  Dot Product4/1 -> [n5cross], Product4/2
  [vr_norm] -> Dot Product4/1
  Constant10/1 -> Dot Product5/2
  Constant11/1 -> Product5/1
  Product5/1 -> [A6cross]
  Dot Product5/1 -> [n6cross], Product5/2
  [vr_norm] -> Dot Product5/1
  Constant12/1 -> Dot Product6/2
  Constant13/1 -> Product6/1
  Product6/1 -> [A7cross]
  Dot Product6/1 -> [n7cross], Product6/2
  [vr_norm] -> Dot Product6/1
  Constant14/1 -> Dot Product7/2
  Constant15/1 -> Product7/1
  Product7/1 -> [A8cross]
  Dot Product7/1 -> [n8cross], Product7/2
  [vr_norm] -> Dot Product7/1
  Constant16/1 -> Dot Product8/2
  Constant17/1 -> Product8/1
  Product8/1 -> [A9cross]
  Dot Product8/1 -> [n9cross], Product8/2
  [vr_norm] -> Dot Product8/1
  Constant18/1 -> Dot Product9/2
  Constant19/1 -> Product9/1
  Product9/1 -> [A10cross]
  Dot Product9/1 -> [n10cross], Product9/2
  [vr_norm] -> Dot Product9/1
  From10/1 -> Mux/1
  From11/1 -> Mux/2
  From12/1 -> Mux/3
  From13/1 -> Mux/4
  From14/1 -> Mux/5
  From15/1 -> Mux/6
  From16/1 -> Mux/7
  From17/1 -> Mux/8
  From18/1 -> Mux/9
  From19/1 -> Mux/10
  [n3cross] -> Mux1/3
  [n6cross] -> Mux1/6
  [n7cross] -> Mux1/7
  [n2cross] -> Mux1/2
  [n10cross] -> Mux1/10
  [n1cross] -> Mux1/1
  [n8cross] -> Mux1/8
  [n9cross] -> Mux1/9
  Mux1/1 -> n_cross/1
  [n4cross] -> Mux1/4
  [n5cross] -> Mux1/5

== system Att_project_simulink/Environment/Air Drag /Air Torque/M1 ==
  F1 : Inport
  n1 : Inport  Port=2
  Constant : Constant  Value=body.r1
  Constant1 : Constant  Value=0
  Cross Product : vrlib/Utilities/Cross Product
  Product : Product
  Switch : Switch  Criteria=u2 > Threshold  SaturateOnIntegerOverflow=off  InputSameDT=off
  M1 : Outport
  wires:
  n1/1 -> Switch/2
  Switch/1 -> Cross Product/1
  Constant/1 -> Cross Product/2
  Constant1/1 -> Switch/3
  Cross Product/1 -> M1/1
  F1/1 -> Product/1
  [A1cross] -> Product/2
  Product/1 -> Switch/1

== system Att_project_simulink/Environment/Air Drag /Air Torque/M10 ==
  F10 : Inport
  n10 : Inport  Port=2
  Constant : Constant  Value=body.r10
  Constant1 : Constant  Value=0
  Cross Product : vrlib/Utilities/Cross Product
  Product : Product
  Switch : Switch  Criteria=u2 > Threshold  SaturateOnIntegerOverflow=off  InputSameDT=off
  M10 : Outport
  wires:
  n10/1 -> Switch/2
  Switch/1 -> Cross Product/1
  Constant/1 -> Cross Product/2
  Cross Product/1 -> M10/1
  Constant1/1 -> Switch/3
  F10/1 -> Product/1
  [A10cross] -> Product/2
  Product/1 -> Switch/1

== system Att_project_simulink/Environment/Air Drag /Air Torque/M2 ==
  F2 : Inport
  n2 : Inport  Port=2
  Constant : Constant  Value=body.r2
  Constant1 : Constant  Value=0
  Cross Product : vrlib/Utilities/Cross Product
  Product : Product
  Switch : Switch  Criteria=u2 > Threshold  SaturateOnIntegerOverflow=off  InputSameDT=off
  M2 : Outport
  wires:
  n2/1 -> Switch/2
  Switch/1 -> Cross Product/1
  Constant/1 -> Cross Product/2
  Cross Product/1 -> M2/1
  Constant1/1 -> Switch/3
  F2/1 -> Product/1
  [A2cross] -> Product/2
  Product/1 -> Switch/1

== system Att_project_simulink/Environment/Air Drag /Air Torque/M3 ==
  F3 : Inport
  n3 : Inport  Port=2
  Constant : Constant  Value=body.r3
  Constant1 : Constant  Value=0
  Cross Product : vrlib/Utilities/Cross Product
  Product : Product
  Switch : Switch  Criteria=u2 > Threshold  SaturateOnIntegerOverflow=off  InputSameDT=off
  M3 : Outport
  wires:
  n3/1 -> Switch/2
  Switch/1 -> Cross Product/1
  Constant/1 -> Cross Product/2
  Cross Product/1 -> M3/1
  Constant1/1 -> Switch/3
  F3/1 -> Product/1
  [A3cross] -> Product/2
  Product/1 -> Switch/1

== system Att_project_simulink/Environment/Air Drag /Air Torque/M4 ==
  F4 : Inport
  n4 : Inport  Port=2
  Constant : Constant  Value=body.r4
  Constant1 : Constant  Value=0
  Cross Product : vrlib/Utilities/Cross Product
  Product : Product
  Switch : Switch  Criteria=u2 > Threshold  SaturateOnIntegerOverflow=off  InputSameDT=off
  M4 : Outport
  wires:
  n4/1 -> Switch/2
  Switch/1 -> Cross Product/1
  Constant/1 -> Cross Product/2
  Cross Product/1 -> M4/1
  Constant1/1 -> Switch/3
  F4/1 -> Product/1
  [A4cross] -> Product/2
  Product/1 -> Switch/1

== system Att_project_simulink/Environment/Air Drag /Air Torque/M5 ==
  F5 : Inport
  n5 : Inport  Port=2
  Constant : Constant  Value=body.r5
  Constant1 : Constant  Value=0
  Cross Product : vrlib/Utilities/Cross Product
  Product : Product
  Switch : Switch  Criteria=u2 > Threshold  SaturateOnIntegerOverflow=off  InputSameDT=off
  M5 : Outport
  wires:
  n5/1 -> Switch/2
  Switch/1 -> Cross Product/1
  Constant/1 -> Cross Product/2
  Cross Product/1 -> M5/1
  Constant1/1 -> Switch/3
  F5/1 -> Product/1
  [A5cross] -> Product/2
  Product/1 -> Switch/1

== system Att_project_simulink/Environment/Air Drag /Air Torque/M6 ==
  F6 : Inport
  n6 : Inport  Port=2
  Constant : Constant  Value=body.r6
  Constant1 : Constant  Value=0
  Cross Product : vrlib/Utilities/Cross Product
  Product : Product
  Switch : Switch  Criteria=u2 > Threshold  SaturateOnIntegerOverflow=off  InputSameDT=off
  M6 : Outport
  wires:
  n6/1 -> Switch/2
  Switch/1 -> Cross Product/1
  Constant/1 -> Cross Product/2
  Cross Product/1 -> M6/1
  Constant1/1 -> Switch/3
  F6/1 -> Product/1
  [A6cross] -> Product/2
  Product/1 -> Switch/1

== system Att_project_simulink/Environment/Air Drag /Air Torque/M7 ==
  F7 : Inport
  n7 : Inport  Port=2
  Constant : Constant  Value=body.r7
  Constant1 : Constant  Value=0
  Cross Product : vrlib/Utilities/Cross Product
  Product : Product
  Switch : Switch  Criteria=u2 > Threshold  SaturateOnIntegerOverflow=off  InputSameDT=off
  M7 : Outport
  wires:
  n7/1 -> Switch/2
  Switch/1 -> Cross Product/1
  Constant/1 -> Cross Product/2
  Cross Product/1 -> M7/1
  Constant1/1 -> Switch/3
  F7/1 -> Product/1
  [A7cross] -> Product/2
  Product/1 -> Switch/1

== system Att_project_simulink/Environment/Air Drag /Air Torque/M8 ==
  F8 : Inport
  n8 : Inport  Port=2
  Constant : Constant  Value=body.r8
  Constant1 : Constant  Value=0
  Cross Product : vrlib/Utilities/Cross Product
  Product : Product
  Switch : Switch  Criteria=u2 > Threshold  SaturateOnIntegerOverflow=off  InputSameDT=off
  M8 : Outport
  wires:
  n8/1 -> Switch/2
  Switch/1 -> Cross Product/1
  Constant/1 -> Cross Product/2
  Cross Product/1 -> M8/1
  Constant1/1 -> Switch/3
  F8/1 -> Product/1
  [A8cross] -> Product/2
  Product/1 -> Switch/1

== system Att_project_simulink/Environment/Air Drag /Air Torque/M9 ==
  F9 : Inport
  n9 : Inport  Port=2
  Constant : Constant  Value=body.r9
  Constant1 : Constant  Value=0
  Cross Product : vrlib/Utilities/Cross Product
  Product : Product
  Switch : Switch  Criteria=u2 > Threshold  SaturateOnIntegerOverflow=off  InputSameDT=off
  M9 : Outport
  wires:
  n9/1 -> Switch/2
  Switch/1 -> Cross Product/1
  Constant/1 -> Cross Product/2
  Cross Product/1 -> M9/1
  Constant1/1 -> Switch/3
  F9/1 -> Product/1
  [A9cross] -> Product/2
  Product/1 -> Switch/1

== matlab function Att_project_simulink/Environment/Air Drag /MATLAB Function1 ==
  data: R input size=1; Rho output size=1
function Rho = Rho_variation(R)
%For interpolation of drag depending on the altitude
R_E=astroConstants(23);
h=R_E+linspace(10,1000,100);
rho = (1e-3) .* [4.02e-04 8.34e-05 1.57e-05 3.18e-06 8.37e-07 2.33e-07 5.86e-08 1.40e-08 2.99e-09 5.17e-10 8.42e-11 1.84e-11 7.36e-12 3.78e-12 2.19e-12 1.37e-12 9.00e-13 6.15e-13 4.32e-13 3.10e-13  2.27e-13 1.68e-13 1.26e-13 9.58e-14 7.35e-14 5.68e-14 4.43e-14 3.48e-14 2.75e-14 2.18e-14   1.74e-14 1.40e-14 1.13e-14 9.10e-15 7.39e-15 6.02e-15 4.92e-15 4.03e-15 3.31e-15 2.72e-15   2.25e-15 1.86e-15 1.54e-15 1.28e-15 1.07e-15 8.89e-16 7.43e-16 6.22e-16 5.22e-16 4.39e-16 3.71e-16 3.13e-16 2.66e-16 2.26e-16 1.93e-16 1.65e-16 1.41e-16 1.22e-16 1.05e-16 9.14e-16 7.96e-17 6.97e-17 6.12e-17 5.41e-17 4.79e-17 4.27e-17 3.82e-17 3.44e-17 3.10e-17 2.82e-17 2.57e-17 2.35e-17 2.16e-17 1.99e-17 1.84e-17 1.71e-17 1.59e-17 1.49e-17 1.39e-17 1.31e-17 1.23e-17 1.16e-17 1.10e-17 1.04e-17 9.86e-18 9.37e-18 8.91e-18 8.48e-18 8.09e-18 7.72e-18  7.37e-18 7.04e-18 6.74e-18 6.45e-18 6.18e-18 5.92e-18 5.68e-18 5.44e-18 5.22e-18 5.02e-18];  
   
%Interpolation
  Rho=interp1(h,rho,R);

== matlab function Att_project_simulink/Environment/Air Drag /MATLAB Function ==
  data: a input; v output; e input; i input; omega input; w input; theta input; mu input
function v =kp2rv(a,e,i,omega,w,theta,mu)
p=a*(1-e^2);
r=p/(1+e*cos(theta));
rpf=r*[cos(theta);sin(theta);0];
v=sqrt(mu/p)*[-sin(theta); e+cos(theta);0];
Rw=[cos(w) sin(w) 0;-sin(w) cos(w) 0; 0 0 1];
Ri=[1 0 0;0 cos(i) sin(i); 0 -sin(i) cos(i)];
Romega=[cos(omega) sin(omega) 0; -sin(omega) cos(omega) 0;0 0 1];
Rge2pf=Rw*Ri*Romega;
Rpf2ge=inv(Rge2pf);
r=Rpf2ge*rpf;
v=(Rpf2ge*v)*1e3;

== matlab function Att_project_simulink/Environment/Magnetif Field Model/MATLAB Function ==
  data: long input; B output; radius input; alpha_G input; lat input; g input; h input; K input; R input; N input
function B = magneticField(long,radius,alpha_G,lat,g,h,K,R,N)
%{  
    Return the magnetic field component in inertial reference frame

%}
theta = (pi/2-lat);     % theta is the colatitude [rad]
alpha = long + alpha_G; 


%% P-dP
% validated through the P and dP tables in "Jeremy Davis, Mathematical Modeling of Earthas Magnetic
% Field, 2004"

%%%%%%%%%%%%%%%%%%%%%%%%%%%%%%%%%%%%%%%%%%%%%%%%%%%%%%%%%%%%%%%%%%%%%%%%%%%%%%%%%%%%%%%%%%%%%%%%
% P_{(n),(m+1)}: 
% given P(a,b) -> n=a, m=b-1
% n from 1 to N
% m from 0 to N
% N order of accuracy
%%%%%%%%%%%%%%%%%%%%%%%%%%%%%%%%%%%%%%%%%%%%%%%%%%%%%%%%%%%%%%%%%%%%%%%%%%%%%%%%%%%%%%%%%%%%%%%%

P = zeros(N,N+1);
dP = zeros(N,N+1);

P_00 = 1;
dP_00 = 0;

P_01 = 0; 
dP_01 = 0;

P(1,1) = cos(theta); % n=1, m=0
dP(1,1) = -sin(theta)*P_00; 

P(1,2) = sin(theta);  % n=1, m=1
dP(1,2) = cos(theta)*P_00;

for i = 2:N % ciclo in n a partire da n=2 a n=N
    for j = 0:i % ciclo in m da m=0 a m=n
        if j == i
        P(i,j+1) = sin(theta)*P(i-1,j);
        dP(i,j+1) = sin(theta)*dP(i-1,j) + cos(theta)*P(i-1,j);
        elseif i < 3
            if j == 0 % n=2, m=0
            P(i,j+1) = cos(theta)*P(i-1,j+1) - K(i,j+1)*P_00;
            dP(i,j+1) = -sin(theta)*P(i-1,j+1) + cos(theta)*dP(i-1,j+1) ...
                - K(i,j+1)*dP_00;
            elseif j == 1 % n=2, m=1
                P(i,j+1) = cos(theta)*P(i-1,j+1) - K(i,j+1)*P_01;
                dP(i,j+1) = -sin(theta)*P(i-1,j+1) + cos(theta)*dP(i-1,j+1)...
                    - K(i,j+1)*dP_01;
            end
        else
            P(i,j+1) = cos(theta)*P(i-1,j+1) - K(i,j+1)*P(i-2,j+1);
            dP(i,j+1) = -sin(theta)*P(i-1,j+1) + cos(theta)*dP(i-1,j+1) ...
                - K(i,j+1)*dP(i-2,j+1);
        end
    end
end

%% Magnetic Field

B_r = 0;
B_th = 0;
B_phi = 0;

%indice i scorre n da 1 a N
%indice j scorre m da 0 a n

for m = 0:N
    for n = 1:N
        if m<=n
            B_r = B_r + (R/radius)^(n+2)*(n+1)*...
                ((g(n,m+1)*cos(m*long) + h(n,m+1)*sin(m*long))*P(n, m+1));
            B_th = B_th + (R/radius)^(n+2)*...
                ((g(n,m+1)*cos(m*long) + h(n,m+1)*sin(m*long))*dP(n, m+1));
            B_phi = B_phi + (R/radius)^(n+2)*...
                (m*(-g(n,m+1)*sin(m*long) + h(n,m+1)*cos(m*long))* P(n, m+1));

        end

    end
end

B_th = -B_th;
B_phi = -B_phi/sin(theta);

B_x = ( B_r*cos(lat) + B_th*sin(lat) ) * cos(alpha) - B_phi*sin(alpha);
B_y = ( B_r*cos(lat) + B_th*sin(lat) ) * sin(alpha) + B_phi*cos(alpha);
B_z = B_r*sin(lat) + B_th*cos(lat);

B = [B_x B_y B_z]';

== matlab function Att_project_simulink/Attitude determination/w_esti/MATLAB Function ==
  data: w input; w_est output
function w_est = fcn(w)


wx_est = w(3,2);

wy_est = w(1,3);

wz_est = w(2,1);

w_est = [wx_est wy_est wz_est]';
